simulink model "vehicle_hostmodel_2023a_RR"  (R2023a)
settings: Solver=VariableStepAuto  StartTime=0  StopTime=1000  FixedStep=0.01  RelTol=1e-3
model workspace (MAT data in the model file):
  finalint = 0
  firstWarning = 1
  originalScenarioChecksum = '114339432DE22364D47BB28FC96DC10C'
undefined symbols (not defined in the file): Acceleration, ActorID, AngularVelocity, curvature, DefaultGear, Defined, DEND_B, DEND_S, DEND_T, direction, DiscIntNeverNeededParam, driving, Ego, gradbp, L, Lane, LF, LR, m, matlabshared, MAX_BRAKE, MAX_STEER, MAX_TORQUE, maxNumActors, MCAR, MIN_BRAKE, MIN_STEER, MIN_TORQUE, n, NUMD_B, NUMD_S, NUMD_T, Pitch, Pose, Position, psi_o, R, Roll, RRdamp, SceneInfo, session, sigbuilder_block, STEER_RATIO, stopSign_ID, Tdead, thetaRefs, TL_ID, TrackWidth, ts, Ts, User, Vdead, Velocity, WB, X_o, xRef2s, Y_o, Yaw, yRef2s
libraries: drivingscenarioandsensors x13, roadrunnerscenario x11, simulink x8, simulink_extras x5, drivingvehiclecontroller x2, trackingutilitieslib x2, robotalgslib x1, mpcadaslib x1, slpidlib x1, drivinglib x1, autolibshared x1, vehdynlibviscommon x1
(part 2 of 4)

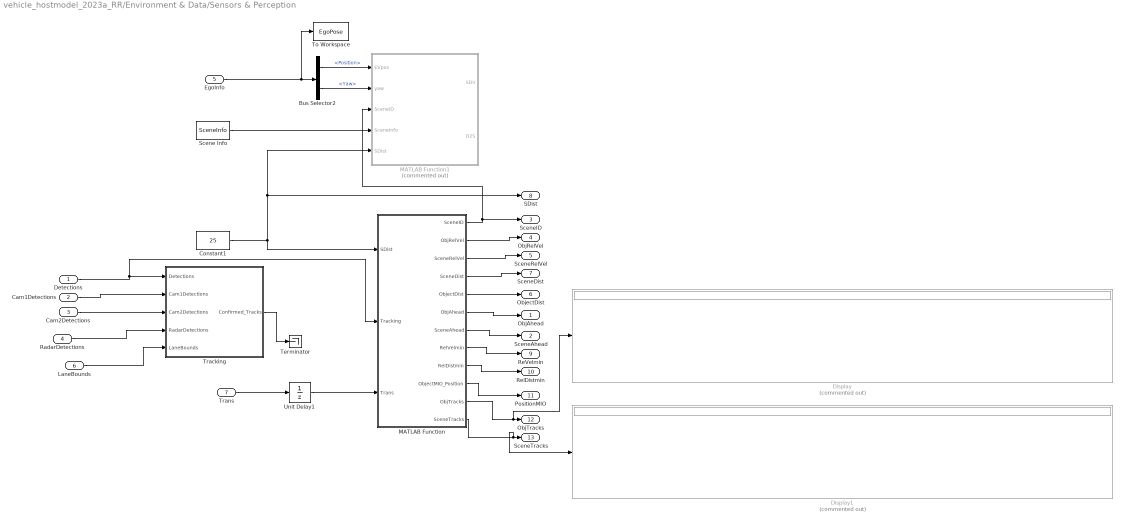
== system vehicle_hostmodel_2023a_RR/Environment & Data/Sensors & Perception ==
  Detections : Inport
  Cam1Detections : Inport  Port=2
  Cam2Detections : Inport  Port=3
  RadarDetections : Inport  Port=4
  EgoInfo : Inport  Port=5
  LaneBounds : Inport  Port=6
  Trans : Inport  Port=7
  Bus Selector2 : BusSelector  OutputSignals=Position,Yaw
  Constant1 : Constant  Value=25
  Display : Display  Commented=on
  Display1 : Display  Commented=on
  MATLAB Function : MATLAB Function  TreatAsAtomicUnit=on
  MATLAB Function1 : MATLAB Function  Commented=on  TreatAsAtomicUnit=on
  Scene Info : Constant  Value=SceneInfo  VectorParams1D=off
  Terminator : Terminator
  To Workspace : ToWorkspace  VariableName=EgoPose  SaveFormat=Timeseries  SampleTime=-1
  Tracking : Subsystem
  Unit Delay1 : UnitDelay  SampleTime=0.05  HasFrameUpgradeWarning=on
  ObjAhead : Outport
  SceneAhead : Outport  Port=2
  SceneID : Outport  Port=3
  ObjRelVel : Outport  Port=4
  SceneRelVel : Outport  Port=5
  ObjectDist : Outport  Port=6
  SceneDist : Outport  Port=7
  SDist : Outport  Port=8
  ReVelmin : Outport  Port=9
  RelDistmin : Outport  Port=10
  PositionMIO : Outport  Port=11
  ObjTracks : Outport  Port=12
  SceneTracks : Outport  Port=13
  wires:
  MATLAB Function/6(ObjAhead) -> ObjAhead/1
  MATLAB Function/5(ObjectDist) -> ObjectDist/1
  MATLAB Function/7(SceneAhead) -> SceneAhead/1
  MATLAB Function/2(ObjRelVel) -> ObjRelVel/1
  EgoInfo/1 -> To Workspace/1, Bus Selector2/1
  Bus Selector2/1 -> MATLAB Function1/1(EVpos)  "<Position>"
  Detections/1 -> MATLAB Function/2(Tracking), Tracking/1(Detections)
  Scene Info/1 -> MATLAB Function1/4(SceneInfo)
  Bus Selector2/2 -> MATLAB Function1/2(yaw)  "<Yaw>"
  Tracking/1(Confirmed_Tracks) -> Terminator/1
  Constant1/1 -> MATLAB Function1/5(SDist), SDist/1, MATLAB Function/1(SDist)
  MATLAB Function/1(SceneID) -> MATLAB Function1/3(SceneID), SceneID/1
  MATLAB Function/4(SceneDist) -> SceneDist/1
  MATLAB Function/3(SceneRelVel) -> SceneRelVel/1
  MATLAB Function/8(RelVelmin) -> ReVelmin/1
  MATLAB Function/9(RelDistmin) -> RelDistmin/1
  Trans/1 -> Unit Delay1/1
  Unit Delay1/1 -> MATLAB Function/3(Trans)
  LaneBounds/1 -> Tracking/5(LaneBounds)
  MATLAB Function/10(ObjectMIO_Position) -> PositionMIO/1
  MATLAB Function/11(ObjTracks) -> Display/1, ObjTracks/1
  MATLAB Function/12(SceneTracks) -> Display1/1, SceneTracks/1
  Cam1Detections/1 -> Tracking/2(Cam1Detections)
  Cam2Detections/1 -> Tracking/3(Cam2Detections)
  RadarDetections/1 -> Tracking/4(RadarDetections)

== system vehicle_hostmodel_2023a_RR/Environment & Data/Subsystem1 ==
  VehFdbk : Inport
  Bus Selector : BusSelector  OutputSignals=InertFrm.Cg.Disp.X,InertFrm.Cg.Disp.Y,InertFrm.Cg.Ang.psi
  Gain1 : Gain  Gain=180/pi
  Mux : Mux  Inputs=3
  Transpose : Math  Operator=transpose  SignedPower=on
  pose : Outport
  wires:
  Mux/1 -> Transpose/1
  VehFdbk/1 -> Bus Selector/1
  Gain1/1 -> Mux/3
  Transpose/1 -> pose/1
  Bus Selector/3 -> Gain1/1  "<psi>"
  Bus Selector/2 -> Mux/2  "<Y>"
  Bus Selector/1 -> Mux/1  "<X>"

== system vehicle_hostmodel_2023a_RR/Environment & Data/Visualisation & Data ==
  note: Load Scenario
  note: Traffic Lights and Stop Signs
  EgoVehStates : Inport
  EgoVelocity : Inport  Port=2
  Ego Acceleration : Inport  Port=3
  Ego Position : Inport  Port=4
  EgoInfo : Inport  Port=5
  Bus Selector : BusSelector  OutputSignals=Actors
  Display : Display
  Display3 : Display
  Lights and Signs ID : Subsystem
  "Positions and States " : Subsystem
  Scenario Reader : drivingscenarioandsensors/Scenario Reader  ScenarioSource=From workspace  ScenarioFileName=\\coeit.osu.edu\home\a\almudhaf.3\Documents\MATLAB\planningControl-Simulation-main\scenarios\BrakingTest.mat  ScenarioVariableName=scenario  OutputCoordinateSystem=Vehicle coordinates  EgoVehicleSource=Input port  EgoVehicleActorID=1  OrientVehiclesOnRoad=on  OutputEgoVehiclePose=on  OutputEgoVehicleState=off  SampleTime=Ts  LaneBoundaryOutput=All lane boundaries  LaneBoundaryDistance=0:0.5:9.5  LaneBoundaryLocation=Center of lane markings  BusNameSource=Auto  BusName=BusActors  BusNumActorsSource=Scenario  BusNumActors=100  BusName2Source=Auto  BusName2=BusLaneBoundaries  BusNumLaneBoundariesSource=Scenario  BusNumLaneBoundaries=10  BusName3Source=Auto  BusName3=BusEgoActor  BusName4Source=Auto  BusName4=BusEgoState  ShowCoordinateLabels=on  SimulateUsing=Interpreted execution
  To Workspace : ToWorkspace  VariableName=SimVel  SampleTime=-1
      settings: Save2DSignal=2-D array (concatenate along first dimension)
  To Workspace1 : ToWorkspace  VariableName=actors  SaveFormat=Timeseries  SampleTime=-1
  To Workspace9 : ToWorkspace  VariableName=SimPos  SampleTime=-1
      settings: Save2DSignal=2-D array (concatenate along first dimension)
  Vehicle To World : drivingscenarioandsensors/Vehicle To World  BusNameSource=Auto  BusName=BusVehicleToWorldActors  SimulateUsing=Interpreted execution
  Visualization : Subsystem
  Actors_VehCoords : Outport
  TL_poses : Outport  Port=2
  actorsinfo : Outport  Port=3
  LaneBounds : Outport  Port=4
  wires:
  Vehicle To World/1 -> To Workspace1/1, actorsinfo/1, Bus Selector/1, Visualization/2(Actors)
  EgoVelocity/1 -> To Workspace/1, Display/1
  Scenario Reader/1 -> Vehicle To World/1, Actors_VehCoords/1
  "Positions and States "/1(TL_poses) -> TL_poses/1, Visualization/1(TL1_poses)
  Lights and Signs ID/1(TL) -> "Positions and States "/2(TL_id)
  Lights and Signs ID/2(Stop_Sign) -> "Positions and States "/3(ss_State)
  "Positions and States "/2(ss_poses) -> Visualization/4(ss1_poses)
  Ego Acceleration/1 -> Display3/1
  Ego Position/1 -> To Workspace9/1
  EgoInfo/1 -> Visualization/3(EgoInfo)
  EgoVehStates/1 -> Vehicle To World/2, Scenario Reader/1
  Bus Selector/1 -> "Positions and States "/1(<Actors>)  "<Actors>"
  Scenario Reader/2 -> LaneBounds/1

== system vehicle_hostmodel_2023a_RR/Reference Data1/Subsystem ==
  In1 : Inport
  Enable : EnablePort
  Step : Step
  Step1 : Step  Time=10
  Sum : Sum  Inputs=|+-
  Out1 : Outport
  wires:
  Sum/1 -> Out1/1
  Step/1 -> Sum/1
  Step1/1 -> Sum/2

== system vehicle_hostmodel_2023a_RR/Reference Data1/Subsystem1 ==
  Integrator : Inport
  enable : Inport  Port=2
  Display : Display
  Subsystem2 : Subsystem
  Subsystem3 : Subsystem
  Switch : Switch  Threshold=1  SaturateOnIntegerOverflow=off  InputSameDT=off
  Ref pose : Outport
  wires:
  enable/1 -> Switch/2
  Integrator/1 -> Subsystem2/1(Integrator), Subsystem3/2(integrator)
  Subsystem2/1(RefPose) -> Display/1, Switch/3
  Subsystem3/1(RefPose) -> Switch/1
  Switch/1 -> Ref pose/1

== system vehicle_hostmodel_2023a_RR/Reference Data1/Subsystem2 ==
  VelFdbk : Inport
  Action Port : ActionPort
  Subsystem : Subsystem
  RefPose : Outport
  DirectionO : Outport  Port=2
  CurvatureO : Outport  Port=3
  WayPoints : Outport  Port=4
  finalint : Outport  Port=5
  wires:
  Subsystem/1(Out1) -> WayPoints/1
  Subsystem/4(DirectionO) -> DirectionO/1
  VelFdbk/1 -> Subsystem/1(In1)
  Subsystem/2(Out2) -> RefPose/1
  Subsystem/3(CurvatureO) -> CurvatureO/1
  Subsystem/5(finalint) -> finalint/1

== system vehicle_hostmodel_2023a_RR/Reference Data1/Subsystem3 ==
  VelFdbk : Inport
  xd : Inport  Port=2
  finalint : Inport  Port=3
  yd : Inport  Port=4
  Action Port : ActionPort
  Subsystem : Subsystem
  RefPose : Outport
  DirectionO : Outport  Port=2
  CurvatureO : Outport  Port=3
  WayPoints : Outport  Port=4
  wires:
  Subsystem/1(Out1) -> WayPoints/1
  Subsystem/4(DirectionO) -> DirectionO/1
  VelFdbk/1 -> Subsystem/1(In1)
  Subsystem/2(Out2) -> RefPose/1
  Subsystem/3(CurvatureO) -> CurvatureO/1
  xd/1 -> Subsystem/2(xd)
  yd/1 -> Subsystem/4(yd)
  finalint/1 -> Subsystem/3(finalint)

== system vehicle_hostmodel_2023a_RR/Subsystem/Function-Call Subsystem ==
  note: put multipler just to change sign to check
  EgoPosition : Inport
  MIOPos : Inport  Port=2
  Road Curvature : Inport  Port=3
  Velocity_Initial_Ego : Inport  Port=4
  MIOVel : Inport  Port=5
  V_desired : Inport  Port=6
  laneL : Inport  Port=7
  laneR : Inport  Port=8
  function : TriggerPort  VariantControl=(inherit)  ShowOutputPort=on
  MATLAB Function1 : MATLAB Function  Commented=on  TreatAsAtomicUnit=on
  MATLAB Function2 : MATLAB Function  TreatAsAtomicUnit=on
  Multiply : Gain  Commented=through  Gain=-1
  Multiply1 : Gain  Gain=-1
  Scope : Scope  NumInputPorts=2
  xd : Outport  InitialOutput=zeros(99,1)
  yd : Outport  Port=2  InitialOutput=zeros(99,1)
  LCinProgress : Outport  Port=3  InitialOutput=0
  wires:
  EgoPosition/1 -> MATLAB Function2/1(EgoPosition), MATLAB Function1/1(EgoPosition)
  MIOPos/1 -> MATLAB Function2/2(MIOPos), MATLAB Function1/2(MIOPos)
  Road Curvature/1 -> MATLAB Function2/3(curvature), MATLAB Function1/3(curvature)
  MIOVel/1 -> MATLAB Function2/4(MIOVel), MATLAB Function1/4(MIOVel)
  Velocity_Initial_Ego/1 -> MATLAB Function2/5(V_i), MATLAB Function1/5(V_i)
  ? -> Scope/1
  ? -> Multiply/1, Scope/2
  V_desired/1 -> MATLAB Function2/8(V_desired), MATLAB Function1/8(V_desired)
  laneL/1 -> MATLAB Function2/6(laneL), MATLAB Function1/6(laneL)
  laneR/1 -> MATLAB Function2/7(laneR), MATLAB Function1/7(laneR)
  Multiply1/1 -> yd/1
  MATLAB Function2/1(xd) -> xd/1
  MATLAB Function2/2(yd) -> Multiply1/1
  MATLAB Function2/3(LCinProgress) -> LCinProgress/1

== system vehicle_hostmodel_2023a_RR/Subsystem/PathPlanner ==
  note: The Path Planning module takes in Trajector generated during Lane change
      | and merges it with current trajectory.
      |
      |
      | If Lane change takes place: Planning module will only work on straight roads.
      |
      | if Lane change doesnt take place: Planning module will work anyway
  CurrentPose : Inport
  xd : Inport  Port=2
  xref : Inport  Port=3
  yref : Inport  Port=4
  yd : Inport  Port=5
  LC : Inport  Port=6
  Cast To Boolean : DataTypeConversion  OutDataTypeStr=boolean  SaturateOnIntegerOverflow=off  RndMeth=Floor
  Delay1 : Delay  DelayLength=1
  Delay2 : Delay  DelayLength=1
  Demux : Demux  Outputs=3
  MATLAB Function3 : MATLAB Function  TreatAsAtomicUnit=on
  MATLAB Function4 : MATLAB Function  TreatAsAtomicUnit=on
  Rate Transition : RateTransition
  Terminator : Terminator
  out : Outport
  check : Outport  Port=2
  dcheck : Outport  Port=3
  wires:
  MATLAB Function3/3(dcheck) -> dcheck/1
  MATLAB Function4/1(Distance) -> Delay1/1
  yd/1 -> MATLAB Function3/4(yd)
  Delay1/1 -> MATLAB Function3/7(d2f)
  CurrentPose/1 -> Demux/1, MATLAB Function4/2(CurrentPose)
  MATLAB Function4/2(point) -> Terminator/1
  MATLAB Function3/1(out) -> MATLAB Function4/1(output), out/1
  xd/1 -> MATLAB Function3/3(xd)
  LC/1 -> MATLAB Function3/5(LC), Delay2/1
  Delay2/1 -> Rate Transition/1
  Demux/2 -> MATLAB Function3/6(current_pos)
  Cast To Boolean/1 -> check/1
  MATLAB Function3/2(check) -> Cast To Boolean/1
  xref/1 -> MATLAB Function3/1(Xref)
  yref/1 -> MATLAB Function3/2(Yref)

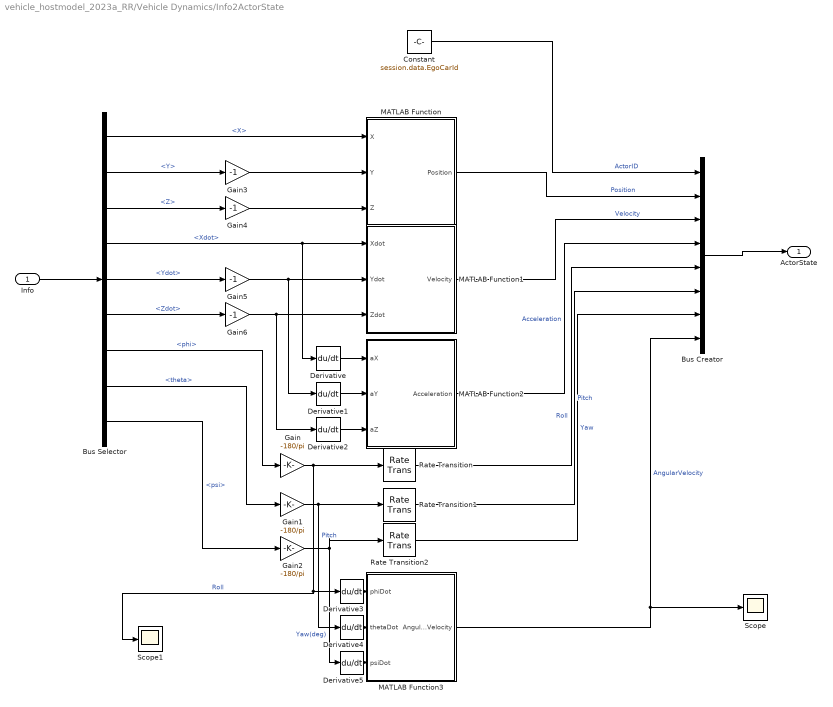
== system vehicle_hostmodel_2023a_RR/Vehicle Dynamics/Info2ActorState ==
  Info : Inport
  Bus Creator : BusCreator  Inputs=ActorID,Position,Velocity,Acceleration,Roll,Pitch,Yaw,AngularVelocity  OutDataTypeStr=Bus: BusActorState  NonVirtualBus=on
  Bus Selector : BusSelector  OutputSignals=InertFrm.Cg.Disp.X,InertFrm.Cg.Disp.Y,InertFrm.Cg.Disp.Z,InertFrm.Cg.Vel.Xdot,InertFrm.Cg.Vel.Ydot,InertFrm.Cg.Vel.Zdot,InertFrm.Cg.Ang.phi,InertFrm.Cg.Ang.theta,InertFrm.Cg.Ang.psi
  Constant : Constant  Value=session.data.EgoCarId  SampleTime=0.05
  Derivative{,1..5} (6 alike) : Derivative
  Gain : Gain  Gain=-180/pi
  Gain1 : Gain  Gain=-180/pi
  Gain2 : Gain  Gain=-180/pi
  Gain{3..6} (4 alike) : Gain  Gain=-1
  MATLAB Function : MATLAB Function  TreatAsAtomicUnit=on  SystemSampleTime=0.05
  MATLAB Function1 : MATLAB Function  TreatAsAtomicUnit=on  SystemSampleTime=0.05
  MATLAB Function2 : MATLAB Function  TreatAsAtomicUnit=on  SystemSampleTime=0.05
  MATLAB Function3 : MATLAB Function  TreatAsAtomicUnit=on  SystemSampleTime=0.05
  Rate Transition : RateTransition  OutPortSampleTime=0.05
  Rate Transition1 : RateTransition  OutPortSampleTime=0.05
  Rate Transition2 : RateTransition  OutPortSampleTime=0.05
  Scope : Scope
  Scope1 : Scope
  ActorState : Outport
  wires:
  Gain/1 -> Scope1/1, Derivative3/1, Rate Transition/1  "Roll"
  Derivative4/1 -> MATLAB Function3/2(thetaDot)
  Bus Selector/2 -> Gain3/1  "<Y>"
  Bus Selector/4 -> Derivative/1, MATLAB Function1/1(Xdot)  "<Xdot>"
  MATLAB Function1/1(Velocity) -> Bus Creator/3  "Velocity"
  MATLAB Function/1(Position) -> Bus Creator/2  "Position"
  Derivative1/1 -> MATLAB Function2/2(aY)
  Bus Selector/5 -> Gain5/1  "<Ydot>"
  Bus Selector/1 -> MATLAB Function/1(X)  "<X>"
  Bus Selector/9 -> Gain2/1  "<psi>"
  Gain2/1 -> Rate Transition2/1, Derivative5/1  "Yaw(deg)"
  Derivative5/1 -> MATLAB Function3/3(psiDot)
  Bus Selector/7 -> Gain/1  "<phi>"
  MATLAB Function2/1(Acceleration) -> Bus Creator/4  "Acceleration"
  Derivative3/1 -> MATLAB Function3/1(phiDot)
  Gain1/1 -> Derivative4/1, Rate Transition1/1  "Pitch"
  Bus Selector/6 -> Gain6/1  "<Zdot>"
  Bus Selector/8 -> Gain1/1  "<theta>"
  MATLAB Function3/1(AngularVelocity) -> Bus Creator/8, Scope/1  "AngularVelocity"
  Bus Selector/3 -> Gain4/1  "<Z>"
  Derivative2/1 -> MATLAB Function2/3(aZ)
  Derivative/1 -> MATLAB Function2/1(aX)
  Info/1 -> Bus Selector/1
  Constant/1 -> Bus Creator/1  "ActorID"
  Bus Creator/1 -> ActorState/1
  Rate Transition/1 -> Bus Creator/5  "Roll"
  Rate Transition1/1 -> Bus Creator/6  "Pitch"
  Rate Transition2/1 -> Bus Creator/7  "Yaw"
  Gain3/1 -> MATLAB Function/2(Y)
  Gain4/1 -> MATLAB Function/3(Z)
  Gain5/1 -> Derivative1/1, MATLAB Function1/2(Ydot)
  Gain6/1 -> Derivative2/1, MATLAB Function1/3(Zdot)

== system vehicle_hostmodel_2023a_RR/Vehicle Dynamics/Subsystem ==
  Gain : Gain  Gain=MAX_TORQUE*0.1
  Gain1 : Gain  Gain=MIN_BRAKE*0.06
  Gain2 : Gain  Gain=MAX_STEER/4.5
  Signal Builder : Subsystem  Tag=STV Subsys  LoadFcn=sigbuilder_block('load');  StartFcn=sigbuilder_block('start');  StopFcn=sigbuilder_block('stop');  ClipboardFcn=sigbuilder_block('clipboard');  mask(Sigbuilder block){tuvar=[0:10]}
      mask help: Simulink:masks:SigbuilderBlock_MD
      mask init:
      | if ~strcmp(get_param(bdroot(gcbh),'SimulationStatus'),'stopped') tuvar = sigbuilder_block('maskInit'); end
      settings: CopyFcn=sigbuilder_block('copy');  DeleteFcn=sigbuilder_block('delete');  ModelCloseFcn=sigbuilder_block('modelClose');  PreSaveFcn=sigbuilder_block('preSave');  PauseFcn=sigbuilder_block('pause');  ContinueFcn=sigbuilder_block('continue');  NameChangeFcn=sigbuilder_block('namechange');  OpenFcn=sigbuilder_block('open',[0 30 960 455.5 ]);  CloseFcn=sigbuilder_block('close');
      mask Display: plot(0, 0, 100, 100,[2, 2, 32, 32, 2], [68, 8, 8, 68, 68],[32, 2], [38, 38], [32, 19, 2],[53, 60, 44], [32, 17, 17, 2],[16, 16, 31, 31]);txt = getActiveGroup(gcbh);text(2, 100, txt,'verticalAlignment', 'top');
  torque_cmd (Nm) : Outport
  brake_cmd (Nm) : Outport  Port=2
  steer_cmd (deg) : Outport  Port=3
  wires:
  Gain2/1 -> steer_cmd (deg)/1  "steer_cmd (deg)"
  Signal Builder/1(Normalized Torque) -> Gain/1
  Signal Builder/2(Normalized Brake) -> Gain1/1
  Signal Builder/3(Normalized Steer) -> Gain2/1  "steer_cmd (deg)"
  Gain1/1 -> brake_cmd (Nm)/1  "brake_cmd (Nm)"
  Gain/1 -> torque_cmd (Nm)/1  "torque_cmd (Nm)"

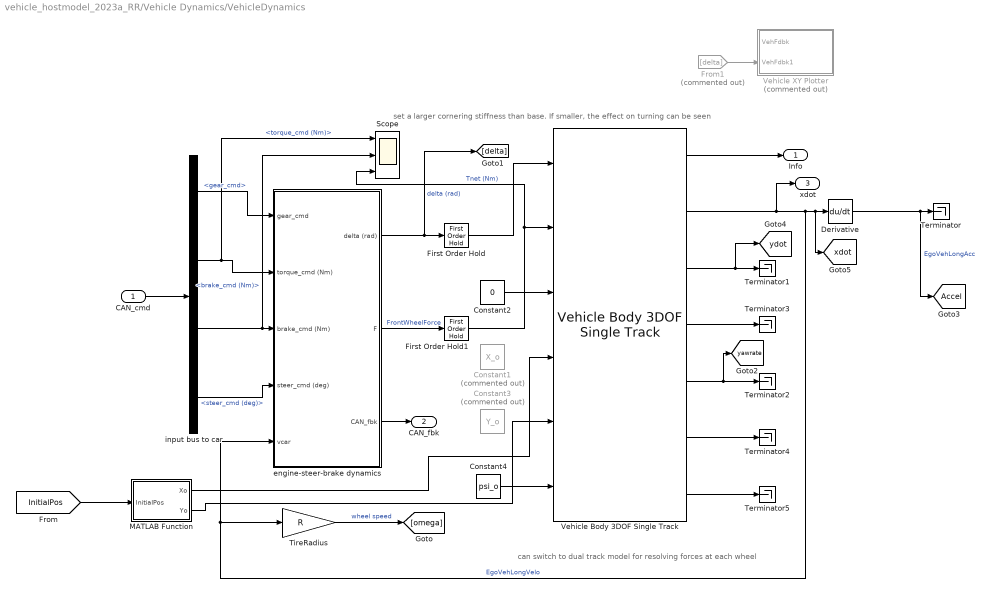
== system vehicle_hostmodel_2023a_RR/Vehicle Dynamics/VehicleDynamics ==
  note: set a larger cornering stiffness than base. If smaller, the effect on turning can be seen
  note: can switch to dual track model for resolving forces at each wheel
  CAN_cmd : Inport
  Constant1 : Constant  Commented=on  Value=X_o
  Constant2 : Constant  Value=0
  Constant3 : Constant  Commented=on  Value=Y_o
  Constant4 : Constant  Value=psi_o
  Derivative : Derivative
  First Order Hold : FirstOrderHold  ErrorTolerance=inf
  First Order Hold1 : FirstOrderHold  ErrorTolerance=inf
  From1 : From  Commented=on  GotoTag=delta
  MATLAB Function : MATLAB Function  TreatAsAtomicUnit=on
  Scope : Scope  NumInputPorts=3
  Terminator{,1..5} (6 alike) : Terminator
  TireRadius : Gain  Gain=R
  Vehicle Body 3DOF Single Track : autolibshared/Vehicle Body 3DOF Single Track  trackMode=Single (bicycle)  inputMode=External longitudinal forces  frontSteerMode=on  rearSteerMode=off  windMode=off  muMode=off  extFMode=off  extMMode=off  htchFMode=off  htchMMode=off  extXo=on  extpsio=on  extxdoto=off  extro=off  extYo=on  extTamb=off  extydoto=off  aMode=2  NF=2  NR=2  m=MCAR  a=LF  b=LR  h=0.35  dh=1  hh=0.2  X_o=InitPosition(1)  xdot_o=InitSpeed  CalphaMode=off  sigmaMode=on  d=0  hl=0  w=[1.4,1.4]  Cy_f=12e3*100  Cy_r=11e3*100  sigma_f=.1  sigma_r=.1  alpha_f_brk=[-.1 .1]  Cy_f_data=[-9e3 9e3]  alpha_r_brk=[-.1 .1]  Cy_r_data=[-9e3 9e3]  Y_o=-InitPosition(2)  ydot_o=0  Izz=2050  psi_o=-InitYaw/180*pi  r_o=0  Af=2  Cd=.3  Cl=.1  Cpm=.1  beta_w=[0:0.01:0.3]  Cs=[0:0.03:0.9]  Cym=[0:0.01:0.3]  Pabs=101325  Tair=273  g=9.81  mu=1  xdot_tol=.01  Fznom=5000  Fxtire_sat=7e4  Fytire_sat=7e4  longOff=0  latOff=0  vertOff=0  wrapAng=off
  Vehicle XY Plotter : Subsystem  Commented=on  mask(Vehicle XY Plotter){a=LF, b=LR, w=TrackWidth, bufferSize=1024, pltDT=.1}
      mask prompts: a "Distance to front axle from CG, a [m]:"; b "Distance to rear axle from CG, b [m]:"; w "Track width, w [m]:"; bufferSize "Path buffer sampe size, bufferSize []:"; pltDT "Plot update rate, pltDT [s]:"
      mask help: This block will display a MATLAB figure which indicates the vehicle path, current position and heading velocity.
      mask TypeOptions a: Vehicle XY Plotter/a
      mask TypeOptions b: Vehicle XY Plotter/b
      mask TypeOptions w: Vehicle XY Plotter/w
      mask TypeOptions bufferSize: Vehicle XY Plotter/bufferSize
  engine-steer-brake dynamics : Subsystem
  input bus to car : BusSelector  OutputSignals=gear_cmd,torque_cmd (Nm),brake_cmd (Nm),steer_cmd (deg)
  Info : Outport
  CAN_fbk : Outport  Port=2  VectorParamsAs1DForOutWhenUnconnected=off
  xdot : Outport  Port=3
  tag scope: Accel=global, xdot=global, yawrate=global, ydot=global
  wires:
  TireRadius/1 -> [omega]  "wheel speed"
  Vehicle Body 3DOF Single Track/1 -> Info/1
  From1/1 -> Vehicle XY Plotter/2(VehFdbk1)
  input bus to car/1 -> engine-steer-brake dynamics/1(gear_cmd)  "<gear_cmd>"
  input bus to car/3 -> Scope/2, engine-steer-brake dynamics/3(brake_cmd (Nm))  "<brake_cmd (Nm)>"
  engine-steer-brake dynamics/1(delta (rad)) -> [delta], First Order Hold/1  "delta (rad)"
  input bus to car/2 -> Scope/1, engine-steer-brake dynamics/2(torque_cmd (Nm))  "<torque_cmd (Nm)>"
  input bus to car/4 -> engine-steer-brake dynamics/4(steer_cmd (deg))  "<steer_cmd (deg)>"
  engine-steer-brake dynamics/3(CAN_fbk) -> CAN_fbk/1
  CAN_cmd/1 -> input bus to car/1
  Constant2/1 -> Vehicle Body 3DOF Single Track/3
  engine-steer-brake dynamics/2(F) -> First Order Hold1/1  "FrontWheelForce"
  First Order Hold/1 -> Vehicle Body 3DOF Single Track/1
  Vehicle Body 3DOF Single Track/2 -> xdot/1, engine-steer-brake dynamics/5(vcar), TireRadius/1, [xdot], Derivative/1  "EgoVehLongVelo"
  Vehicle Body 3DOF Single Track/3 -> [ydot], Terminator1/1
  Vehicle Body 3DOF Single Track/4 -> Terminator3/1
  Vehicle Body 3DOF Single Track/5 -> [yawrate], Terminator2/1
  Vehicle Body 3DOF Single Track/6 -> Terminator4/1
  Vehicle Body 3DOF Single Track/7 -> Terminator5/1
  Derivative/1 -> [Accel], Terminator/1  "EgoVehLongAcc"
  First Order Hold1/1 -> Scope/3, Vehicle Body 3DOF Single Track/2  "Tnet (Nm)"
  Constant4/1 -> Vehicle Body 3DOF Single Track/6
  [InitialPos] -> MATLAB Function/1(InitialPos)
  MATLAB Function/1(Xo) -> Vehicle Body 3DOF Single Track/4
  MATLAB Function/2(Yo) -> Vehicle Body 3DOF Single Track/5

== system vehicle_hostmodel_2023a_RR/Controllers/Lateral Controllers1/Pure Pursuit Controller1 ==
  note: The subsystem implements a Pure Pursuit controller. The "Pure Pursuit" block calculates the target direction and the "Wheel Steering Angle Formulation" block calculates the wheel steering angle.
  Pose : Inport
  Waypoints : Inport  Port=2
  Pure Pursuit : robotalgslib/Pure Pursuit  DesiredLinearVelocity=0.1  MaxAngularVelocity=1.0  LookaheadDistance=6  TargetDirPort=on  SimulateUsing=Interpreted execution
  Terminator6 : Terminator
  Terminator7 : Terminator
  Wheel Steering Angle Formulation : Subsystem  mask{L=L, ld=10}
      mask prompts: L "Bicycle length"; ld "Lookahead distance"
      mask TypeOptions L: Bicycle length/Value
      mask TypeOptions ld: Lookahead distance/Value
      mask Display:
      | image("GeometryMask.png")
      | port_label('input', 1, 'alpha')
      | port_label('output', 1, 'delta')
  delta : Outport
  wires:
  Wheel Steering Angle Formulation/1(Al) -> delta/1
  Pure Pursuit/3 -> Wheel Steering Angle Formulation/1(alpha)
  Pure Pursuit/2 -> Terminator7/1
  Pose/1 -> Pure Pursuit/1
  Pure Pursuit/1 -> Terminator6/1
  Waypoints/1 -> Pure Pursuit/2

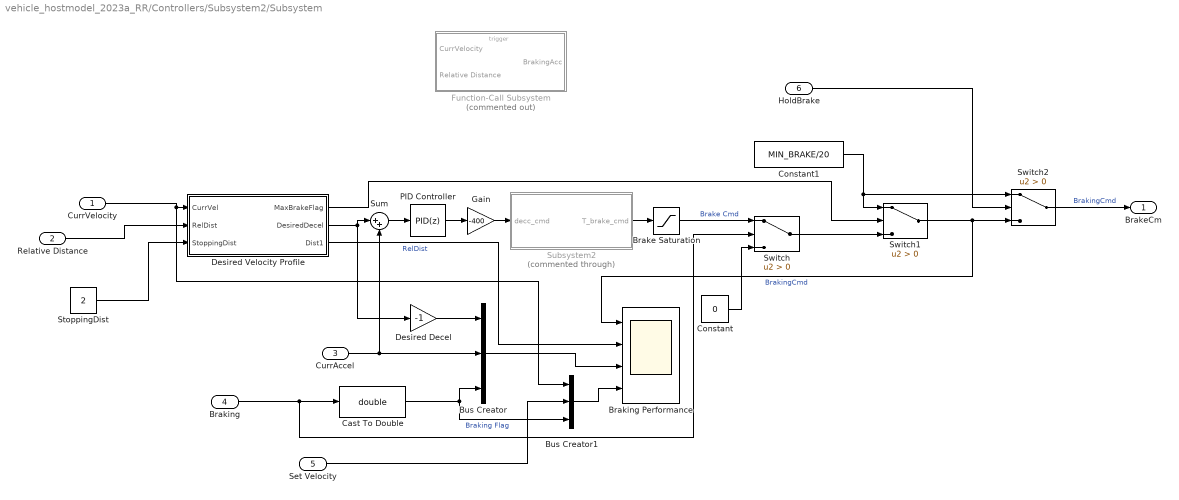
== system vehicle_hostmodel_2023a_RR/Controllers/Subsystem2/Subsystem ==
  CurrVelocity : Inport
  Relative Distance : Inport  Port=2
  CurrAccel : Inport  Port=3
  "Braking " : Inport  Port=4
  Set Velocity : Inport  Port=5
  HoldBrake : Inport  Port=6
  Brake Saturation : Saturate  UpperLimit=MAX_BRAKE  LowerLimit=MIN_BRAKE
  Braking Performance : Scope  NumInputPorts=4
  Bus Creator : BusCreator  Inputs=3
  Bus Creator1 : BusCreator  Inputs=3
  Cast To Double : DataTypeConversion  OutDataTypeStr=double  SaturateOnIntegerOverflow=off  RndMeth=Floor
  Constant : Constant  Value=0
  Constant1 : Constant  Value=MIN_BRAKE/20
  Desired Decel : Gain  Gain=-1
  Desired Velocity Profile : MATLAB Function  TreatAsAtomicUnit=on
  Function-Call Subsystem : Subsystem  Commented=on  TreatAsAtomicUnit=on
  Gain : Gain  Gain=-400
  PID Controller : slpidlib/PID Controller  Controller=PID  Form=Parallel  TimeDomain=Discrete-time  UseExternalTs=off  SampleTime=-1  IntegratorMethod=Forward Euler  FilterMethod=Forward Euler  ControllerParametersSource=internal  P=0.05*20  I=0.01*10  UseKiTs=off  D=0  N=100  UseFilter=on  TunerSelectOption=Transfer Function Based (PID Tuner App)  InitialConditionSource=internal  InitialConditionForIntegrator=0  InitialConditionForFilter=0  DifferentiatorICPrevScaledInput=0  ExternalReset=none  TrackingMode=off  Kt=1  LimitOutput=off  SatLimitsSource=internal  UpperSaturationLimit=inf  LowerSaturationLimit=-inf  LinearizeAsGain=on  AntiWindupMode=none  Kb=1  LimitIntegrator=off  UpperIntegratorSaturationLimit=inf  LowerIntegratorSaturationLimit=-inf  POutMin=[]  POutMax=[]  IOutMin=[]  IOutMax=[]  DOutMin=[]  DOutMax=[]  NOutMin=[]  NOutMax=[]  SumOutMin=[]  SumOutMax=[]  SaturationOutMin=[]  SaturationOutMax=[]  PParamMin=[]  PParamMax=[]  IParamMin=[]  IParamMax=[]  DParamMin=[]  DParamMax=[]  NParamMin=[]  NParamMax=[]  KbParamMin=[]  KbParamMax=[]  KtParamMin=[]  KtParamMax=[]  KbOutMin=[]  KbOutMax=[]  KtOutMin=[]  KtOutMax=[]  IntegratorOutMin=[]  IntegratorOutMax=[]  FilterOutMin=[]  FilterOutMax=[]  SumI1OutMin=[]  SumI1OutMax=[]  SumI2OutMin=[]  SumI2OutMax=[]  SumI3OutMin=[]  SumI3OutMax=[]  SumI4OutMin=[]  SumI4OutMax=[]  SumDOutMin=[]  SumDOutMax=[]  DifferentiatorOutMin=[]  DifferentiatorOutMax=[]  FilterDiffOutCoefMin=[]  FilterDiffOutCoefMax=[]  ReciprocalOutMin=[]  ReciprocalOutMax=[]  SumDenOutMin=[]  SumDenOutMax=[]  SumNumOutMin=[]  SumNumOutMax=[]  DivideOutMin=[]  DivideOutMax=[]  UdiffTsProdOutMin=[]  UdiffTsProdOutMax=[]  NTsProdOutMin=[]  NTsProdOutMax=[]  UintegralTsProdOutMin=[]  UintegralTsProdOutMax=[]  UngainTsProdOutMin=[]  UngainTsProdOutMax=[]  ClampingZeroOutDataTypeStr=Inherit: Inherit via back propagation  ClampingZeroOutMin=[]  ClampingZeroOutMax=[]  FilterDenConstantOutDataTypeStr=Inherit: Inherit via back propagation  FilterDenConstantOutMin=[]  FilterDenConstantOutMax=[]  PCopyOutDataTypeStr=Inherit: Inherit via back propagation  PCopyOutMin=[]  PCopyOutMax=[]  NCopyOutDataTypeStr=Inherit: Inherit via back propagation  NCopyOutMin=[]  NCopyOutMax=[]  IntegratorContinuousStateAttributes=''  IntegratorStateMustResolveToSignalObject=off  IntegratorRTWStateStorageClass=Auto  FilterContinuousStateAttributes=''  FilterStateMustResolveToSignalObject=off  FilterRTWStateStorageClass=Auto  ParallelPVariant=InternalParameters  IdealPVariant=Disabled  IVariant=InternalParameters  DVariant=InternalParameters  IntegratorVariant=Discrete  SatVariant=Disabled  AWVariant=Passthrough  PCopyVariant=Disabled  TRVariant=Disabled  FdbkBlocksVariant=Forward  IdealPFdbkVariant=Disabled  SatFdbkVariant=Disabled  DerivativeFilterVariant=ForwardEulerFilter  NVariant=InternalParameters  NCopyVariant=Disabled  FilterICVariant=InternalICsFilter  IntegratorICVariant=InternalICs  ExternalResetVariant=Disabled  TRSumVariant=Passthrough  SumFdbkVariant=Disabled  SumVariant=Sum_PID  TsampFilterVariant=InternalTs  TsampNgainVariant=Passthrough  TsampIntegralVariant=Disabled_SignalSpec  ExternalSaturationOutDataTypeStr=Inherit: Same as second input
  StoppingDist : Constant  Value=2
  Subsystem2 : Subsystem  Commented=through
  Sum : Sum  Inputs=|++
  Switch : Switch  Criteria=u2 > Threshold  SaturateOnIntegerOverflow=off  InputSameDT=off
  Switch1 : Switch  Criteria=u2 > Threshold  SaturateOnIntegerOverflow=off  InputSameDT=off
  Switch2 : Switch  Criteria=u2 > Threshold  SaturateOnIntegerOverflow=off  InputSameDT=off
  BrakeCm : Outport
  wires:
  PID Controller/1 -> Gain/1
  Relative Distance/1 -> Desired Velocity Profile/2(RelDist)
  CurrVelocity/1 -> Bus Creator1/1, Desired Velocity Profile/1(CurrVel)
  Sum/1 -> PID Controller/1
  Subsystem2/1(T_brake_cmd) -> Brake Saturation/1
  Desired Velocity Profile/2(DesiredDecel) -> Sum/1, Desired Decel/1
  "Braking "/1 -> Cast To Double/1, Switch/2
  Brake Saturation/1 -> Switch/1  "Brake Cmd"
  CurrAccel/1 -> Bus Creator/2, Sum/2
  Gain/1 -> Subsystem2/1(decc_cmd)
  Desired Decel/1 -> Bus Creator/1
  Constant/1 -> Switch/3
  Switch1/1 -> Switch2/3, Braking Performance/1  "BrakingCmd"
  Bus Creator/1 -> Braking Performance/3
  Cast To Double/1 -> Bus Creator1/3, Bus Creator/3  "Braking Flag"
  Desired Velocity Profile/3(Dist1) -> Braking Performance/2  "RelDist"
  Switch/1 -> Switch1/3
  Constant1/1 -> Switch2/1, Switch1/1
  Desired Velocity Profile/1(MaxBrakeFlag) -> Switch1/2
  Bus Creator1/1 -> Braking Performance/4
  Set Velocity/1 -> Bus Creator1/2
  StoppingDist/1 -> Desired Velocity Profile/3(StoppingDist)
  HoldBrake/1 -> Switch2/2
  Switch2/1 -> BrakeCm/1  "BrakingCmd"

== system vehicle_hostmodel_2023a_RR/Controllers/Subsystem2/Subsystem1 ==
  acc_cmd : Inport
  decc_cmd : Inport  Port=2
  Brake Saturation : Saturate  UpperLimit=MAX_BRAKE  LowerLimit=MIN_BRAKE
  Constant : Constant  Value=0
  Subsystem2 : Subsystem
  Switch : Switch  Criteria=u2 > Threshold  Threshold=500  SaturateOnIntegerOverflow=off  InputSameDT=off
  Switch1 : Switch  Criteria=u2 > Threshold  Threshold=-500  SaturateOnIntegerOverflow=off  InputSameDT=off
  Throttle Saturation : Saturate  UpperLimit=MAX_TORQUE  LowerLimit=MIN_TORQUE
  second-order low-pass brake model1 : DiscreteTransferFcn  Commented=through  Numerator=DEND_B  Denominator=NUMD_B  SampleTime=ts
  second-order low-pass torque model : DiscreteTransferFcn  Commented=through  Numerator=DEND_T  Denominator=NUMD_T  SampleTime=ts
  torque_cm : Outport
  brake_cm : Outport  Port=2
  wires:
  Subsystem2/1(T_eng_cmd) -> second-order low-pass torque model/1
  acc_cmd/1 -> Subsystem2/1(acc_cmd)
  second-order low-pass brake model1/1 -> Brake Saturation/1
  Subsystem2/2(brake_cmd) -> second-order low-pass brake model1/1
  decc_cmd/1 -> Subsystem2/2(decc_cmd)
  second-order low-pass torque model/1 -> Throttle Saturation/1
  Throttle Saturation/1 -> Switch/2, Switch/1
  Switch/1 -> torque_cm/1
  Brake Saturation/1 -> Switch1/2, Switch1/3
  Switch1/1 -> brake_cm/1
  Constant/1 -> Switch/3, Switch1/1

== system vehicle_hostmodel_2023a_RR/Environment & Data/Roadrunner Port/BusActorPose To BusVehiclePose ==
  BusActorPose : Inport
  Bus Creator : BusCreator  Inputs=7  OutDataTypeStr=Bus: BusVehiclePose  NonVirtualBus=on
      settings: InheritFromInputs=off
  Bus Selector : BusSelector  OutputSignals=ActorID,Position,Velocity,Roll,Pitch,Yaw,AngularVelocity
  BusVehiclePose : Outport
  wires:
  BusActorPose/1 -> Bus Selector/1
  Bus Selector/1 -> Bus Creator/1  "<ActorID>"
  Bus Selector/2 -> Bus Creator/2  "<Position>"
  Bus Selector/4 -> Bus Creator/4  "<Roll>"
  Bus Selector/5 -> Bus Creator/5  "<Pitch>"
  Bus Selector/6 -> Bus Creator/6  "<Yaw>"
  Bus Selector/7 -> Bus Creator/7  "<AngularVelocity>"
  Bus Selector/3 -> Bus Creator/3  "<Velocity>"
  Bus Creator/1 -> BusVehiclePose/1

== system vehicle_hostmodel_2023a_RR/Environment & Data/Roadrunner Port/Calculate Norm ==
  Lateral Velocity : Inport
  Longitudinal Velocity : Inport  Port=2
  Add : Sum
  Math Function : Math  Operator=square
  Math Function1 : Math  Operator=square
  Sqrt : Sqrt
  Speed : Outport
  wires:
  Add/1 -> Sqrt/1
  Math Function1/1 -> Add/2
  Math Function/1 -> Add/1
  Sqrt/1 -> Speed/1
  Lateral Velocity/1 -> Math Function/1
  Longitudinal Velocity/1 -> Math Function1/1

== system vehicle_hostmodel_2023a_RR/Environment & Data/Roadrunner Port/ENU to NWD ==
  RR Position : Inport
  2D RefWaypoints : MATLAB Function  TreatAsAtomicUnit=on
  Display : Display  Commented=on
  Display1 : Display
  Display2 : Display  Commented=on
  Display4 : Display
  Display5 : Display
  Gain : Gain  Gain=-1
  MATLAB Function : MATLAB Function  TreatAsAtomicUnit=on
  MATLAB Function1 : MATLAB Function  Commented=on  TreatAsAtomicUnit=on
  MATLAB Function2 : MATLAB Function  TreatAsAtomicUnit=on
  Matrix Concatenate : Concatenate  NumInputs=3  Mode=Multidimensional array  ConcatenateDimension=2
  Selector : Selector  NumberOfDimensions=2  InputPortWidth=3  IndexOptions=Select all,Index vector (dialog)  Indices=[1 3],1  OutputSizes=1,1
  Selector1 : Selector  NumberOfDimensions=2  InputPortWidth=3  IndexOptions=Select all,Index vector (dialog)  Indices=[1 3],2  OutputSizes=1,1
  Selector2 : Selector  NumberOfDimensions=2  InputPortWidth=3  IndexOptions=Select all,Index vector (dialog)  Indices=[1 3],3  OutputSizes=1,1
  Cuboid Position : Outport
  Trajectory Destination : Outport  Port=2
  Waypts_traj : Outport  Port=3
  Trajectory Start : Outport  Port=4
  wires:
  Gain/1 -> Matrix Concatenate/2
  Selector1/1 -> Matrix Concatenate/1
  Selector2/1 -> Matrix Concatenate/3
  Selector/1 -> Gain/1
  RR Position/1 -> Selector/1, Selector1/1, Selector2/1
  Matrix Concatenate/1 -> MATLAB Function2/1(u), MATLAB Function1/1(traj), 2D RefWaypoints/1(u), MATLAB Function/1(traj), Cuboid Position/1
  MATLAB Function/1(destination_traj) -> Trajectory Destination/1
  MATLAB Function1/1(trajectory_way) -> Display1/1
  MATLAB Function2/1(y) -> Display/1
  MATLAB Function2/2(y1) -> Display2/1
  2D RefWaypoints/1(y) -> Waypts_traj/1
  MATLAB Function/3(Initial_traj) -> Trajectory Start/1

== system vehicle_hostmodel_2023a_RR/Environment & Data/Roadrunner Port/Initiaal State ==
  VehicleRuntime : Inport
  SteerCmd : Inport  Port=2
  Info : Inport  Port=3
  CurrVelocity : Inport  Port=4
  yawrate : Inport  Port=5
  Constant5 : Constant
  Initialize State : Subsystem
  Pack Current States : Subsystem
  CurrVehicleInfo : Outport
  wires:
  Constant5/1 -> Pack Current States/6(Direction)
  Initialize State/1(InitialState) -> Pack Current States/5(egoInitialState)
  VehicleRuntime/1 -> Initialize State/1(VehicleRuntime)
  yawrate/1 -> Pack Current States/4(CurrYawRate)
  CurrVelocity/1 -> Pack Current States/3(CurrVelocity)
  Info/1 -> Pack Current States/2(Info)
  SteerCmd/1 -> Pack Current States/1(CurrSteer)
  Pack Current States/1(CurrVehicleInfo) -> CurrVehicleInfo/1

== system vehicle_hostmodel_2023a_RR/Environment & Data/Roadrunner Port/NWD to ENU ==
  Cuboid Pose : Inport
  Gain : Gain  Commented=through  Gain=180/pi
  Gain1 : Gain  Gain=-1
  Matrix Concatenate : Concatenate  NumInputs=3  Mode=Multidimensional array  ConcatenateDimension=2
  Selector : Selector  InputPortWidth=3  IndexOptions=Index vector (dialog)  Indices=3  OutputSizes=1
  Selector1 : Selector  InputPortWidth=3  IndexOptions=Index vector (dialog)  Indices=1  OutputSizes=1
  Selector2 : Selector  InputPortWidth=3  IndexOptions=Index vector (dialog)  Indices=2  OutputSizes=1
  RR Pose : Outport
  wires:
  Matrix Concatenate/1 -> RR Pose/1
  Selector2/1 -> Gain1/1
  Selector1/1 -> Matrix Concatenate/2
  Selector/1 -> Gain/1
  Cuboid Pose/1 -> Selector1/1, Selector/1, Selector2/1
  Gain1/1 -> Matrix Concatenate/1
  Gain/1 -> Matrix Concatenate/3

== system vehicle_hostmodel_2023a_RR/Environment & Data/Roadrunner Port/Pack Actor Pose ==
  CurrPose : Inport
  CurrSpeed : Inport  Port=2
  VehicleRuntime : Inport  Port=3
  Assign : BusAssignment  AssignedSignals=Pose,Velocity
  Bus Selector : BusSelector  OutputSignals=ActorRuntime
  Pose Generation : MATLAB Function  TreatAsAtomicUnit=on
  Selector : Selector  InputPortWidth=3  IndexOptions=Index vector (dialog)  Indices=3  OutputSizes=1
  Velocity XYZ Components : MATLAB Function  TreatAsAtomicUnit=on
  Ego Pose : Outport
  wires:
  Velocity XYZ Components/1(velocity) -> Assign/3  "Velocity"
  Pose Generation/1(currPose) -> Assign/2  "Pose"
  CurrPose/1 -> Selector/1, Pose Generation/1(pose)
  Selector/1 -> Velocity XYZ Components/1(yaw)
  CurrSpeed/1 -> Velocity XYZ Components/2(speed)
  VehicleRuntime/1 -> Bus Selector/1
  Bus Selector/1 -> Assign/1  "<ActorRuntime>"
  Assign/1 -> Ego Pose/1

== system vehicle_hostmodel_2023a_RR/Environment & Data/Sensors & Perception/Tracking ==
  Detections : Inport
  Cam1Detections : Inport  Port=2
  Cam2Detections : Inport  Port=3
  RadarDetections : Inport  Port=4
  LaneBounds : Inport  Port=5
  Camera : drivingscenarioandsensors/Vision Detection Generator  SensorIndex=2  DetectorOutput=Objects only  UpdateInterval=0.01  LaneUpdateInterval=0.1  SensorLocation=[1.9 0.5]  Height=1.1  Yaw=45  Pitch=0  Roll=0  BusNameSource=Auto  BusName=BusObjectDetections  BusName2Source=Auto  BusName2=BusLaneDetections  MaxNumDetectionsSource=Property  MaxNumDetections=10  MaxNumLanesSource=Property  MaxNumLanes=30  DetectionCoordinates=Ego Cartesian  SimulateUsing=Interpreted execution  MaxRange=150  BoundingBoxAccuracy=1  ProcessNoiseIntensity=1  MaxSpeed=100  MaxAllowedOcclusion=0.99  MinObjectImageSize=[2 2]  DetectionProbability=1  FalsePositivesPerImage=0  MinLaneImageSize=[20 3]  LaneBoundaryAccuracy=3  HasNoise=off  InitialSeedSource=Repeatable  InitialSeed=0  UsedSeed=0  ActorProfilesSource=MATLAB expression  ActorProfilesParameters=driving.internal.ActorProfilesParameters  ActorProfilesExpression=actorProfiles  Intrinsics=driving.internal.cameraIntrinsics('FocalLength',[200 800],'PrincipalPoint',[320 240],'ImageSize',[640 480],'RadialDistortion',[0 0],'TangentialDistortion',[0 0],'Skew',0)
  Camera1 : drivingscenarioandsensors/Vision Detection Generator  SensorIndex=3  DetectorOutput=Objects only  UpdateInterval=0.01  LaneUpdateInterval=0.1  SensorLocation=[1.9 -0.5]  Height=1.1  Yaw=-45  Pitch=0  Roll=0  BusNameSource=Auto  BusName=BusObjectDetections  BusName2Source=Auto  BusName2=BusLaneDetections  MaxNumDetectionsSource=Property  MaxNumDetections=10  MaxNumLanesSource=Property  MaxNumLanes=30  DetectionCoordinates=Ego Cartesian  SimulateUsing=Interpreted execution  MaxRange=150  BoundingBoxAccuracy=1  ProcessNoiseIntensity=1  MaxSpeed=100  MaxAllowedOcclusion=0.99  MinObjectImageSize=[2 2]  DetectionProbability=1  FalsePositivesPerImage=0  MinLaneImageSize=[20 3]  LaneBoundaryAccuracy=3  HasNoise=off  InitialSeedSource=Repeatable  InitialSeed=0  UsedSeed=0  ActorProfilesSource=MATLAB expression  ActorProfilesParameters=driving.internal.ActorProfilesParameters  ActorProfilesExpression=actorProfiles  Intrinsics=driving.internal.cameraIntrinsics('FocalLength',[200 800],'PrincipalPoint',[320 240],'ImageSize',[640 480],'RadialDistortion',[0 0],'TangentialDistortion',[0 0],'Skew',0)
  Detection Concatenation : trackingutilitieslib/Detection Concatenation  NumInputs=3  BusNameSource=Auto  BusName=Detections  SimulateUsing=Interpreted execution
  Display : Display
  Display1 : Display
  Driving Radar Data Generator : drivingscenarioandsensors/Driving Radar Data Generator  SensorIndex=1  UpdateRate=100  MountingLocation=[ 3.4, 0, 0.2 ]  MountingAngles=[0 0 0]  HasElevation=on  HasRangeRate=on  HasNoise=off  HasFalseAlarms=on  HasOcclusion=on  MaxNumReportsSource=Property  MaxNumReports=50  TargetReportFormat=Clustered detections  DetectionCoordinates=Body  TrackCoordinates=Body  BusNameSource=Auto  BusName=BusDrivingRadarDataGenerator  AzimuthResolution=3  ElevationResolution=3  RangeResolution=2.5  RangeRateResolution=0.5  AzimuthBiasFraction=0.1  ElevationBiasFraction=0.1  RangeBiasFraction=0.05  RangeRateBiasFraction=0.05  FieldOfView=[ 180, 6 ]  RangeLimits=[ 0, 150 ]  RangeRateLimits=[ -100, 100 ]  DetectionProbability=1  FalseAlarmRate=1e-06  ReferenceRange=100  ReferenceRCS=0  CenterFrequency=77e9  FilterInitializationFcn=initcvekf  ConfirmationThreshold=[2 3]  DeletionThreshold=[5 5]  InitialSeedSource=Repeatable  InitialSeed=0  UsedSeed=matlabshared.tracking.internal.SimulinkUtilities.seedManager(gcb)  ProfilesSource=MATLAB expression  ProfilesParameters=driving.internal.ActorProfilesRadarParameters  ProfilesExpression=actorProfiles
  MATLAB Function : MATLAB Function  TreatAsAtomicUnit=on
  Multi-Object Tracker : drivinglib/Multi-Object Tracker  TrackerIndex=uint32( 0 )  FilterInitializationFcn=helperInitSimulinkDemoFilter  AssignmentThreshold=30  ConfirmationThreshold=[ 2, 3 ]  DeletionThreshold=[ 6, 6 ]  MaxNumTracks=20  MaxNumSensors=20  OOSMHandling=Neglect  StateParametersSimulink=struct  HasStateParametersInput=off  TimeInputSource=Auto  HasCostMatrixInput=off  HasDetectableTrackIDsInput=off  BusNameSource=Auto  BusName=BusMultiObjectTracker  TentativeTracksOutputPort=off  AllTracksOutputPort=off  SimulateUsing=Interpreted execution
  Subsystem1 : Subsystem  Commented=on
  Terminator : Terminator
  Confirmed_Tracks : Outport
  wires:
  Detections/1 -> Driving Radar Data Generator/1, Camera1/1, Camera/1
  Detection Concatenation/1 -> Multi-Object Tracker/1
  LaneBounds/1 -> Terminator/1
  Multi-Object Tracker/1 -> Confirmed_Tracks/1, MATLAB Function/1(u)
  MATLAB Function/1(y) -> Display/1
  Camera1/1 -> Detection Concatenation/1  "Camera Detections"
  Camera/1 -> Detection Concatenation/2  "Camera Detections"
  MATLAB Function/2(y1) -> Display1/1
  Driving Radar Data Generator/1 -> Detection Concatenation/3

== system vehicle_hostmodel_2023a_RR/Environment & Data/Visualisation & Data/Lights and Signs ID ==
  Constant : Constant  Value=TL_ID
  Constant1 : Constant  Value=stopSign_ID
  TL : Outport
  Stop_Sign : Outport  Port=2
  wires:
  Constant/1 -> TL/1
  Constant1/1 -> Stop_Sign/1

== system vehicle_hostmodel_2023a_RR/Environment & Data/Visualisation & Data/Positions and States  ==
  note: Stop Sign positon
  note: Traffic Light Position and State
  <Actors> : Inport
  TL_id : Inport  Port=2
  ss_State : Inport  Port=3
  MATLAB Function1 : MATLAB Function  TreatAsAtomicUnit=on
  MATLAB Function2 : MATLAB Function  TreatAsAtomicUnit=on
  Traffic Light Sensor : Subsystem  mask{TrafficLightSensorModeSelection=Cycle}
      mask prompts: TrafficLightSensorModeSelection "Traffic Light Sensor Mode:"
      mask TypeOptions TrafficLightSensorModeSelection: Steady Green | Steady Red | Cycle
      mask DialogControl DescTextVar Prompt: Simulate a traffic light sensor.
  TL_poses : Outport
  ss_poses : Outport  Port=2
  wires:
  <Actors>/1 -> MATLAB Function2/1(Actors), MATLAB Function1/1(Actors)
  ss_State/1 -> MATLAB Function2/2(ss_State)
  TL_id/1 -> Traffic Light Sensor/1(TL_id)
  Traffic Light Sensor/1(TL_State) -> MATLAB Function1/2(TL_State)  "TL_State"
  MATLAB Function2/1(ss_poses) -> ss_poses/1
  MATLAB Function1/1(TL_poses) -> TL_poses/1

== system vehicle_hostmodel_2023a_RR/Environment & Data/Visualisation & Data/Visualization ==
  note: Visualization
  TL1_poses : Inport
  Actors : Inport  Port=2
  EgoInfo : Inport  Port=3
  ss1_poses : Inport  Port=4
  Visualization : MATLABSystem  System=TL_vis
      mask Type: TL_vis
      mask Display:
      | disp('TL_vis');
      | port_label('input',1,'TL');
      | port_label('input',2,'TargetPoses');
      | port_label('input',3,'EgoInfo');
      | port_label('input',4,'SS');
  wires:
  EgoInfo/1 -> Visualization/3
  Actors/1 -> Visualization/2  "target_vehicle_poses"
  TL1_poses/1 -> Visualization/1
  ss1_poses/1 -> Visualization/4

== system vehicle_hostmodel_2023a_RR/Reference Data1/Subsystem1/Subsystem2 ==
  Integrator : Inport
  Subsystem : Subsystem
  RefPose : Outport
  DirectionO : Outport  Port=2
  CurvatureO : Outport  Port=3
  WayPoints : Outport  Port=4
  finalint : Outport  Port=5
  wires:
  Subsystem/1(Out1) -> WayPoints/1
  Subsystem/4(DirectionO) -> DirectionO/1
  Subsystem/2(Out2) -> RefPose/1
  Subsystem/3(CurvatureO) -> CurvatureO/1
  Subsystem/5(finalint) -> finalint/1
  Integrator/1 -> Subsystem/1(Integrator)

== system vehicle_hostmodel_2023a_RR/Reference Data1/Subsystem1/Subsystem3 ==
  xd : Inport
  integrator : Inport  Port=2
  yd : Inport  Port=3
  Subsystem : Subsystem
  RefPose : Outport
  DirectionO : Outport  Port=2
  CurvatureO : Outport  Port=3
  WayPoints : Outport  Port=4
  wires:
  Subsystem/1(Out1) -> WayPoints/1
  Subsystem/4(DirectionO) -> DirectionO/1
  Subsystem/2(Out2) -> RefPose/1
  Subsystem/3(CurvatureO) -> CurvatureO/1
  xd/1 -> Subsystem/1(xd)
  yd/1 -> Subsystem/2(yd)
  integrator/1 -> Subsystem/3(Integrator)

== system vehicle_hostmodel_2023a_RR/Reference Data1/Subsystem2/Subsystem ==
  note: Select method to calculate theta
  In1 : Inport
  Curvature : Lookup_n-D  NumberOfTableDimensions=1  BreakpointsForDimension1=gradbp  Table=curvature  InternalRulePriority=Speed  RndMeth=Simplest
  Direction : Lookup_n-D  NumberOfTableDimensions=1  BreakpointsForDimension1=gradbp  Table=direction  InternalRulePriority=Speed  RndMeth=Simplest
  Discrete-Time Integrator : DiscreteIntegrator  SampleTime=-1  ICPrevOutput=DiscIntNeverNeededParam  ICPrevScaledInput=DiscIntNeverNeededParam
  From Workspace1 : FromWorkspace  VariableName=yRef2  SampleTime=-1
  From Workspace2 : FromWorkspace  VariableName=xRef2  SampleTime=-1
  From Workspace3 : FromWorkspace  VariableName=gradbp  SampleTime=-1
  Matrix Concatenate : Concatenate  Mode=Multidimensional array  ConcatenateDimension=2
  Mux : Mux  Inputs=3
  Switch Case : SwitchCase
  Theta : Subsystem  Variant=on  VariantControlMode=label  LabelModeActiveChoice=thetaLookUpTable
  X Ref : Lookup_n-D  NumberOfTableDimensions=1  BreakpointsForDimension1=gradbp  Table=xRef2s  InternalRulePriority=Speed  RndMeth=Simplest
  Y Ref : Lookup_n-D  NumberOfTableDimensions=1  BreakpointsForDimension1Source=Input port  BreakpointsForDimension1=gradbp  TableSource=Input port  Table=yRef2s  InternalRulePriority=Speed  RndMeth=Simplest
      settings: InputPortMap=u0,p221,p5
  Out1 : Outport
  Out2 : Outport  Port=2
  CurvatureO : Outport  Port=3
  DirectionO : Outport  Port=4
  finalint : Outport  Port=5
  tag scope: xRef=global, yRef=global
  wires:
  Direction/1 -> DirectionO/1
  Discrete-Time Integrator/1 -> finalint/1, Curvature/1, Direction/1, Theta/3(dis), Y Ref/1, X Ref/1
  Y Ref/1 -> Theta/1(y), Mux/2, [yRef]
  Theta/1(theta) -> Mux/3
  X Ref/1 -> Theta/2(x), Mux/1, [xRef]
  Matrix Concatenate/1 -> Out1/1
  Curvature/1 -> CurvatureO/1
  Mux/1 -> Out2/1
  From Workspace1/1 -> Y Ref/2, Matrix Concatenate/2
  From Workspace2/1 -> Matrix Concatenate/1
  In1/1 -> Discrete-Time Integrator/1
  From Workspace3/1 -> Y Ref/3

== system vehicle_hostmodel_2023a_RR/Reference Data1/Subsystem3/Subsystem ==
  note: Select method to calculate theta
  In1 : Inport
  xd : Inport  Port=2
  finalint : Inport  Port=3
  yd : Inport  Port=4
  Add Constant : Bias  Bias=8  SaturateOnIntegerOverflow=off
  Curvature : Lookup_n-D  NumberOfTableDimensions=1  BreakpointsForDimension1=gradbp  Table=curvature  InternalRulePriority=Speed  RndMeth=Simplest
  Direction : Lookup_n-D  NumberOfTableDimensions=1  BreakpointsForDimension1=gradbp  Table=direction  InternalRulePriority=Speed  RndMeth=Simplest
  Discrete-Time Integrator : DiscreteIntegrator  InitialConditionSource=external  InitialCondition=finalint  SampleTime=-1  ICPrevOutput=DiscIntNeverNeededParam  ICPrevScaledInput=DiscIntNeverNeededParam
  From Workspace1 : FromWorkspace  VariableName=yRef2  SampleTime=-1
  From Workspace2 : FromWorkspace  VariableName=xRef2  SampleTime=-1
  From Workspace3 : FromWorkspace  VariableName=gradbp  SampleTime=-1
  Goto : Goto  Commented=on  GotoTag=xRef  TagVisibility=global
  Goto1 : Goto  Commented=on  GotoTag=yRef  TagVisibility=global
  Matrix Concatenate : Concatenate  Mode=Multidimensional array  ConcatenateDimension=2
  Mux : Mux  Inputs=3
  Theta : Subsystem  Variant=on  VariantControlMode=label  LabelModeActiveChoice=thetaLookUpTable
  X Ref : Lookup_n-D  NumberOfTableDimensions=1  BreakpointsForDimension1Source=Input port  BreakpointsForDimension1=gradbp  TableSource=Input port  Table=xRef2s  InternalRulePriority=Speed  RndMeth=Simplest
      settings: InputPortMap=u0,p221,p5
  Y Ref : Lookup_n-D  NumberOfTableDimensions=1  BreakpointsForDimension1Source=Input port  BreakpointsForDimension1=gradbp  TableSource=Input port  Table=yRef2s  InternalRulePriority=Speed  RndMeth=Simplest
      settings: InputPortMap=u0,p221,p5
  Out1 : Outport
  Out2 : Outport  Port=2
  CurvatureO : Outport  Port=3
  DirectionO : Outport  Port=4
  wires:
  Direction/1 -> DirectionO/1
  Discrete-Time Integrator/1 -> Curvature/1, Direction/1, Theta/3(dis), Y Ref/1, X Ref/1
  Theta/1(theta) -> Mux/3
  Matrix Concatenate/1 -> Out1/1
  Curvature/1 -> CurvatureO/1
  Mux/1 -> Out2/1
  From Workspace1/1 -> Add Constant/1, Matrix Concatenate/2
  From Workspace2/1 -> X Ref/2, Matrix Concatenate/1
  In1/1 -> Discrete-Time Integrator/1
  From Workspace3/1 -> Y Ref/3, X Ref/3
  X Ref/1 -> Theta/2(x), Mux/1
  finalint/1 -> Discrete-Time Integrator/2
  Add Constant/1 -> Y Ref/2
  Y Ref/1 -> Theta/1(y), Mux/2

== system vehicle_hostmodel_2023a_RR/Vehicle Dynamics/Subsystem/Signal Builder ==
  Demux : Demux  Tag=STV Demux  Outputs=3
      settings: DisplayOption=none
  FromWs : FromWorkspace  Tag=STV FromWs  VariableName=tuvar
      SigBuilderData=|
      | common.afterFinalStr = 'Extrapolate'
      | common.sampleTime = 0
      | dataSet.timeRange = [0 3.5]
      | dataSet.name = 'DriveAndTurn'
      | sbobj.Groups.Name = 'DriveAndTurn'
      | sbobj.Groups.Signals(1).Name = 'Normalized Torque'
      | sbobj.Groups.Signals(1).XData = [0 1 1 2 2 3.5]
      | sbobj.Groups.Signals(1).YData = [1 1 0 0 1 1]
      | sbobj.Groups.Signals(2).Name = 'Normalized Brake'
      | sbobj.Groups.Signals(2).XData = [0 1 1 2 2 3.5]
      | sbobj.Groups.Signals(2).YData = [0 0 1 1 0 0]
      | sbobj.Groups.Signals(3).Name = 'Normalized Steer'
      | sbobj.Groups.Signals(3).XData = [0 0.5 0.6 1.02 1.02 2 2.5 3 3.5]
      | sbobj.Groups.Signals(3).YData = [-0.02 -0.02 -0.02 -0.3 -1.02 -0.92 -0.34 0.14 0.22]
      | sbobj.Groups.TimeRange = [0 3.5]
  Normalized Torque : Outport  Tag=STV Outport
  Normalized Brake : Outport  Tag=STV Outport  Port=2
  Normalized Steer : Outport  Tag=STV Outport  Port=3
  wires:
  FromWs/1 -> Demux/1
  Demux/1 -> Normalized Torque/1
  Demux/2 -> Normalized Brake/1
  Demux/3 -> Normalized Steer/1

== system vehicle_hostmodel_2023a_RR/Vehicle Dynamics/VehicleDynamics/Vehicle XY Plotter ==
  VehFdbk : Inport
  VehFdbk1 : Inport  Port=2
  Bus Selector1 : BusSelector  OutputSignals=InertFrm.Cg.Ang.phi,InertFrm.Cg.Ang.theta,InertFrm.Cg.Ang.psi  OutputAsBus=on
  Bus Selector3 : BusSelector  OutputSignals=InertFrm.Geom.Disp.X,InertFrm.Geom.Disp.Y,InertFrm.Geom.Disp.Z  OutputAsBus=on
  Bus Selector4 : BusSelector  OutputSignals=InertFrm.Cg.Vel.Xdot,InertFrm.Cg.Vel.Ydot  OutputAsBus=on
  Bus to Vector : BusToVector
  Bus to Vector1 : BusToVector
  Bus to Vector2 : BusToVector
  Constant4 : Constant  Value=0
  Ground : Ground
  Rate Transition{1..2,5..6} (4 alike) : RateTransition  OutPortSampleTime=pltDT
  Vector Concatenate : Concatenate
  Vector Concatenate1 : Concatenate  NumInputs=4
  Vehicle XY Plotter : vehdynlibviscommon/Vehicle XY Plotter  w=w  a=a  b=b  figBorder=2000  bufferSize=bufferSize  extStats=off  extTireF=off
  wires:
  Bus to Vector2/1 -> Rate Transition1/1  "InertCGDisp"
  Rate Transition5/1 -> Vehicle XY Plotter/1
  Bus Selector4/1 -> Bus to Vector1/1
  Rate Transition1/1 -> Vehicle XY Plotter/2
  Rate Transition6/1 -> Vehicle XY Plotter/3
  Vector Concatenate/1 -> Rate Transition6/1  "InertCGVel"
  Bus Selector1/1 -> Bus to Vector2/1
  Bus to Vector/1 -> Rate Transition5/1  "InertCGDisp"
  Bus Selector3/1 -> Bus to Vector/1
  Bus to Vector1/1 -> Vector Concatenate/1
  Ground/1 -> Vector Concatenate/2
  VehFdbk/1 -> Bus Selector1/1, Bus Selector4/1, Bus Selector3/1
  Rate Transition2/1 -> Vehicle XY Plotter/4
  Constant4/1 -> Vector Concatenate1/4, Vector Concatenate1/3
  VehFdbk1/1 -> Vector Concatenate1/2, Vector Concatenate1/1  "delta"
  Vector Concatenate1/1 -> Rate Transition2/1  "delta"
